simulink model "coordinated_turn_roll_v1"  (R2022b)
settings: Solver=VariableStepAuto  StartTime=0.0  StopTime=10.0  RelTol=1e-3
settings Model: Creator=Tamer  LastModifiedBy=Tamer
settings SolverCC: ZeroCrossControl=DisableAll  AlgebraicLoopSolver=TrustRegion
settings DataIOCC: SaveOutput=off  SaveTime=off
settings DebuggingCC: UnconnectedInputMsg=warning  UnconnectedOutputMsg=warning  UnconnectedLineMsg=warning  SFMachineParentedDataDiag=warning
settings ModelReferenceCC: EnableRefExpFcnMdlSchedulingChecks=on
settings GRTTargetCC: CombineOutputUpdateFcns=off  MatFileLogging=off

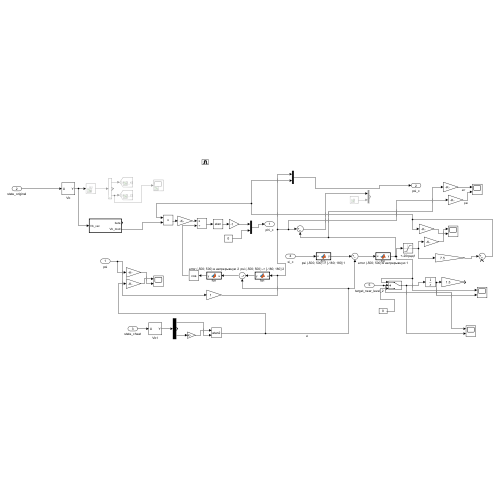
[thumbnail: Simulink's stored preview of the top-level diagram]
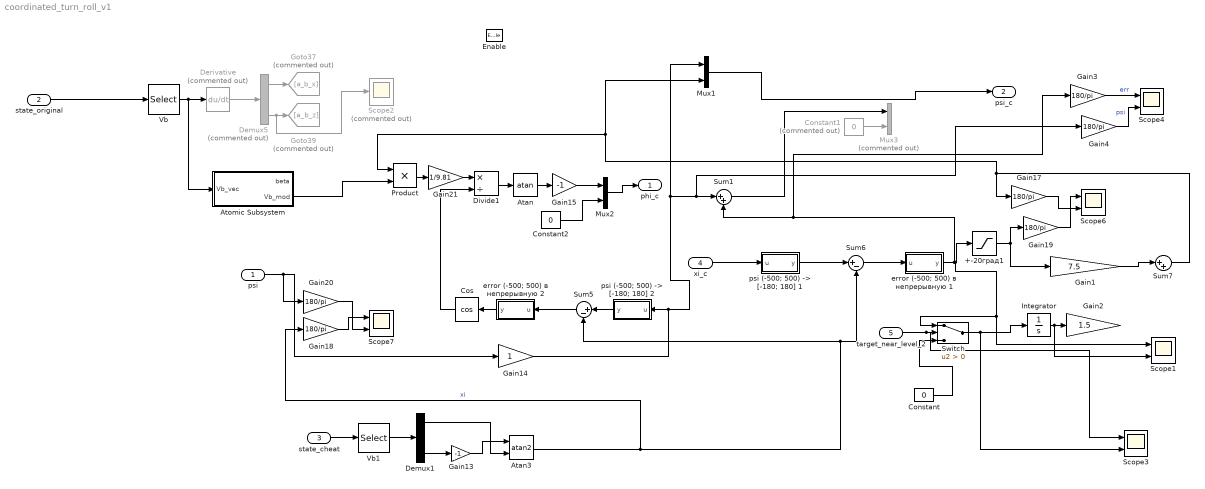
== system coordinated_turn_roll_v1 ==
  psi : Inport
  state_original : Inport  Port=2
  state_cheat : Inport  Port=3
  xi_c : Inport  Port=4
  target_near_level_2 : Inport  Port=5  OutDataTypeStr=boolean
  Enable : EnablePort
  +-20град1 : Saturate  UpperLimit=deg2rad(20)  LowerLimit=-deg2rad(20)
  Atan : Trigonometry  Operator=atan
  Atan3 : Trigonometry  Operator=atan2
  Atomic Subsystem : Subsystem  TreatAsAtomicUnit=on
  Constant : Constant  Value=0
  Constant1 : Constant  Commented=on  Value=0
  Constant2 : Constant  Value=0
  Cos : Trigonometry  Operator=cos
  Demux1 : Demux  Outputs=3
  Demux5 : Demux  Commented=on  Outputs=3
  Derivative : Derivative  Commented=on
  Divide1 : Product  Inputs=*/
  Gain1 : Gain  Gain=7.5
  Gain13 : Gain  Gain=-1
  Gain14 : Gain
  Gain15 : Gain  Gain=-1
  Gain{3..4,17..20} (6 alike) : Gain  Gain=180/pi
  Gain2 : Gain  Gain=1.5
  Gain21 : Gain  Gain=1/9.81
  Goto37 : Goto  Commented=on  GotoTag=a_b_x
  Goto39 : Goto  Commented=on  GotoTag=a_b_z
  Integrator : Integrator
  Mux1 : Mux  Inputs=2
  Mux2 : Mux  Inputs=2
  Mux3 : Mux  Commented=on  Inputs=2
  Product : Product
  Scope{1,3..4,6..7} (5 alike) : Scope  NumInputPorts=2
  Scope2 : Scope  Commented=on
  Sum1 : Sum  Inputs=|++
  Sum5 : Sum  Inputs=|+-
  Sum6 : Sum  Inputs=|+-
  Sum7 : Sum  Inputs=|++
  Switch : Switch  Criteria=u2 > Threshold  SaturateOnIntegerOverflow=off  InputSameDT=off
  Vb : Selector  InputPortWidth=12  IndexOptions=Index vector (dialog)  Indices=[4:6]  OutputSizes=1
  Vb1 : Selector  InputPortWidth=15  IndexOptions=Index vector (dialog)  Indices=[4:6]  OutputSizes=1
  error (-500; 500) в непрерывную 1 : MATLAB Function  TreatAsAtomicUnit=on
  error (-500; 500) в непрерывную 2 : MATLAB Function  TreatAsAtomicUnit=on
  "psi (-500; 500) -> [-180; 180] 1" : MATLAB Function  TreatAsAtomicUnit=on
  "psi (-500; 500) -> [-180; 180] 2" : MATLAB Function  TreatAsAtomicUnit=on
  phi_c : Outport
  psi_c : Outport  Port=2
  wires:
  Derivative/1 -> Demux5/1
  Vb/1 -> Atomic Subsystem/1(Vb_vec), Derivative/1
  Demux5/1 -> Goto37/1
  state_original/1 -> Vb/1
  Demux5/3 -> Scope2/1, Goto39/1
  Vb1/1 -> Demux1/1
  Gain14/1 -> Gain4/1, Sum1/1, Mux1/1, "psi (-500; 500) -> [-180; 180] 2"/1(u)
  Atan/1 -> Gain15/1
  +-20град1/1 -> Gain1/1, Gain19/1
  Gain19/1 -> Scope6/1
  psi/1 -> Gain20/1, Gain14/1
  Sum7/1 -> Mux1/2, Product/1, Gain17/1
  Gain17/1 -> Scope6/2
  state_cheat/1 -> Vb1/1
  Demux1/3 -> Gain13/1
  Atan3/1 -> Sum6/2, Sum5/2, Gain18/1  "xi"
  Gain18/1 -> Scope7/1
  Gain20/1 -> Scope7/2
  Gain13/1 -> Atan3/1
  Demux1/1 -> Atan3/2
  Product/1 -> Gain21/1
  Cos/1 -> Divide1/2
  Gain21/1 -> Divide1/1
  Divide1/1 -> Atan/1
  Gain1/1 -> Sum7/1
  error (-500; 500) в непрерывную 1/1(y) -> Scope1/1, Switch/1, +-20град1/1, Gain3/1, Sum1/2
  Sum6/1 -> error (-500; 500) в непрерывную 1/1(u)
  "psi (-500; 500) -> [-180; 180] 1"/1(y) -> Sum6/1
  error (-500; 500) в непрерывную 2/1(y) -> Cos/1
  Sum5/1 -> error (-500; 500) в непрерывную 2/1(u)
  Atomic Subsystem/2(Vb_mod) -> Product/2
  xi_c/1 -> "psi (-500; 500) -> [-180; 180] 1"/1(u)
  "psi (-500; 500) -> [-180; 180] 2"/1(y) -> Sum5/1
  Gain15/1 -> Mux2/1
  Mux2/1 -> phi_c/1
  Constant2/1 -> Mux2/2
  Integrator/1 -> Scope1/2, Gain2/1
  Switch/1 -> Scope3/2, Integrator/1
  Constant/1 -> Switch/3
  Mux1/1 -> psi_c/1
  Constant1/1 -> Mux3/2
  Sum1/1 -> Mux3/1
  Gain3/1 -> Scope4/1  "err"
  Gain4/1 -> Scope4/2  "psi"
  target_near_level_2/1 -> Scope3/1, Switch/2

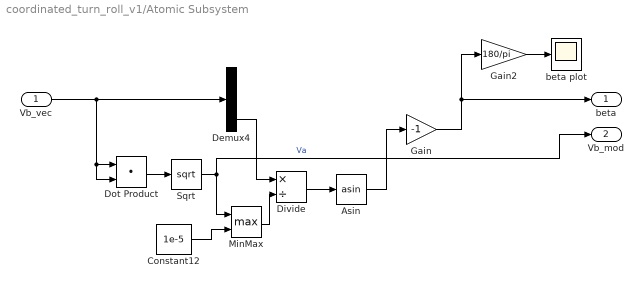
== system coordinated_turn_roll_v1/Atomic Subsystem ==
  Vb_vec : Inport
  Asin : Trigonometry  Operator=asin
  Constant12 : Constant  Value=1e-5
  Demux4 : Demux  Outputs=3
  Divide : Product  Inputs=*/
  Dot Product : DotProduct  OutDataTypeStr=Inherit: Inherit via internal rule
  Gain : Gain  Gain=-1
  Gain2 : Gain  Gain=180/pi
  MinMax : MinMax  Function=max  Inputs=2
  Sqrt : Sqrt
  beta plot : Scope
  beta : Outport
  Vb_mod : Outport  Port=2
  wires:
  Asin/1 -> Gain/1
  Demux4/3 -> Divide/1
  Constant12/1 -> MinMax/2
  Gain/1 -> beta/1, Gain2/1
  Sqrt/1 -> Vb_mod/1, MinMax/1  "Va"
  Vb_vec/1 -> Demux4/1, Dot Product/2, Dot Product/1
  Divide/1 -> Asin/1
  MinMax/1 -> Divide/2
  Dot Product/1 -> Sqrt/1
  Gain2/1 -> beta plot/1

== matlab function coordinated_turn_roll_v1/psi (-500; 500) -> [-180; 180] 1 ==
  data: u input; y output
function y = fcn(u)

y = u - 2*pi*sign(u)*(abs(u) > pi);

== matlab function coordinated_turn_roll_v1/error (-500; 500) в непрерывную 1 ==
  data: u input; y output
function y = fcn(u)

y = u + 2*pi*sign(pi-u).*(abs(u)>pi);

== matlab function coordinated_turn_roll_v1/error (-500; 500) в непрерывную 2 ==
  data: u input; y output
function y = fcn(u)

y = u + 2*pi*sign(pi-u).*(abs(u)>pi);

== matlab function coordinated_turn_roll_v1/psi (-500; 500) -> [-180; 180] 2 ==
  data: u input; y output
function y = fcn(u)

y = u - 2*pi*sign(u)*(abs(u) > pi);
